simulink model "generate_elbow_motion"  (R2020b)
settings: Solver=FixedStepDiscrete  StartTime=0.0  StopTime=inf  FixedStep=0.001  RelTol=1e-3  EnableMultiTasking=on
PreLoadFcn:
  | demos_common_configs();
libraries: franka_simulink_library_misc x5, franka_simulink_library x4, simulink x1
settings Model: SimulationMode=external  ExtModeTrigDuration=10000  Creator=vasi_ko  LastModifiedBy=kvasios
settings DataIOCC: LimitDataPoints=on  SaveFormat=Array  ReturnWorkspaceOutputs=off
settings OptimizationCC: DefaultParameterBehavior=Inlined  EnhancedBackFolding=on  PassReuseOutputArgsAs=Individual arguments  ZeroExternalMemoryAtStartup=off  ZeroInternalMemoryAtStartup=off  OptimizeBlockOrder=speed  DifferentSizesBufferReuse=on  OptimizationCustomize=off  EfficientTunableParamExpr=on
settings DebuggingCC: SolverPrmCheckMsg=warning  ParameterTunabilityLossMsg=error  SFUnexpectedBacktrackingDiag=warning  SFNoUnconditionalDefaultTransitionDiag=warning  SFExecutionAtInitializationDiag=none  ArithmeticOperatorsInVariantConditions=warning
settings HardwareCC: ProdBitPerLong=64  ProdHWDeviceType=Intel->x86-64 (Linux 64)
settings ModelReferenceCC: PropagateSignalLabelsOutOfModel=off
settings SFSimCC: SimUseLocalCustomCode=off  MATLABDynamicMemAlloc=off  CustomCodeUndefinedFunction=UseInterfaceOnly  SimTargetLang=C++
settings RTWCC: Description=Embedded Coder  SystemTargetFile=franka_emika_panda.tlc  GenCodeOnly=on  TemplateMakefile=ert_default_tmf  RTWVerbose=off  RTWUseLocalCustomCode=off  Toolchain=Franka Simulink | gmake (64-bit linux)  BuildConfiguration=Faster Runs  IncludeHyperlinkInReport=on  TargetLang=C++
settings CodeAppCC: ForceParamTrailComments=on  IgnoreCustomStorageClasses=off  OperatorAnnotations=on  SimulinkDataObjDesc=on  SFDataObjDesc=on  InsertBlockDesc=on
settings STFCustomTargetCC: TargetLangStandard=C99 (ISO)  MultiwordLength=256  GenerateSampleERTMain=on  ModelReferenceCompliant=off  ConcurrentExecutionCompliant=off  CombineOutputUpdateFcns=on  ERTCustomFileBanners=on  SupportNonInlinedSFcns=off  RemoveResetFunc=on  MATLABClassNameForMDSCustomization=Simulink.SoftwareTarget.ERTCustomization  GRTInterface=off  UseToolchainInfoCompliant=on  SystemTargetFile=franka_emika_panda.tlc
settings ERTTargetCC: TargetLangStandard=C99 (ISO)  GenerateSampleERTMain=on  ModelReferenceCompliant=off  ParMdlRefBuildCompliant=off  CompOptLevelCompliant=off  ConcurrentExecutionCompliant=off  SupportContinuousTime=on  ModelStepFunctionPrototypeControlCompliant=off  InlinedParameterPlacement=NonHierarchical  ERTCustomFileTemplate=franka_emika_panda_file_process.tlc
settings ConfigComp: CovMetricSettings=dw  CovSaveCumulativeToWorkspaceVar=on  CovSaveSingleToWorkspaceVar=on  CovExternalEMLEnable=off  CovSFcnEnable=off

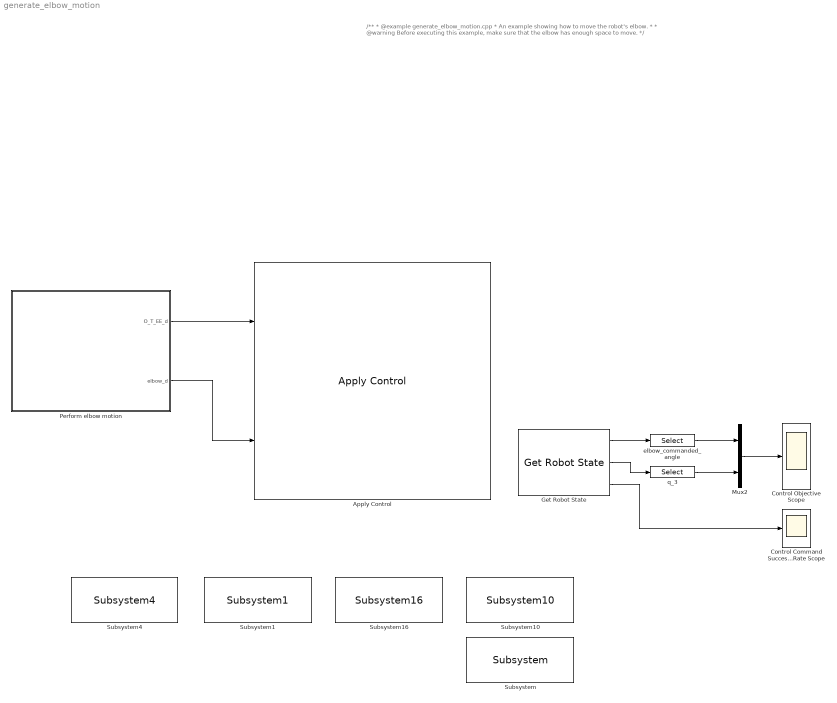
== system generate_elbow_motion ==
  note: /**
      |  * @example generate_elbow_motion.cpp
      |  * An example showing how to move the robot's elbow.
      |  *
      |  * @warning Before executing this example, make sure that the elbow has enough space to move.
      |  */
  Apply Control : franka_simulink_library/Apply Control  robot_ip=robot_ip  gripper_attached=off  control_mode=Cartesian Pose - Internal Controller Mode  controller_choice=Joint Impedance Controller  elbow_control=on  collision_thresholds=[25.0, 25.0, 22.0, 20.0, 19.0, 17.0, 14.0,35.0, 35.0, 32.0, 30.0, 29.0, 27.0, 24.0,25.0, 25.0, 22.0, 20.0, 19.0, 17.0, 14.0,35.0, 35.0, 32.0, 30.0, 29.0, 27.0, 24.0,30.0, 30.0, 30.0, 25.0, 25.0, 25.0,40.0, 40.0, 40.0, 35.0, 35.0, 35.0,30.0, 30.0, 30.0, 25.0, 25.0, 25.0,40.0, 40.0, 40.0, 35.0, 35.0, 35.0]  joint_impedance=[3000, 3000, 3000, 2500, 2500, 2000, 2000]  cartesian_impedance=cartesian_impedance  load_inertia=load_inertia  EE_T_K=EE_T_K  init_joint_configuration_req=on  init_joint_configuration=q_init
      settings: SourceProductName=Franka Emika
  Control Command Success Rate Scope : Scope
  Control Objective Scope : Scope
  Get Robot State : franka_simulink_library/Get Robot State  robot_ip=robot_ip  signals_requested='elbow_c q control_command_success_rate'
      settings: SourceProductName=Franka Emika
  Mux2 : Mux  Inputs=2
  Perform elbow motion : Subsystem
      mask Display:
      | pos = get_param(gcb, 'Position');
      | width = pos(3) - pos(1);
      | x = [0:width];
      | y = sin(x/180*pi);
      | % Parameters 'm' and 'b' must be defined in 'Parameters & Dialog' pane.
      | plot(cos(x/180*pi*0.5), sin(x/180*pi*0.5));
      | 
      | port_label('output',1,'O_T_EE_d');
      | port_label('output',2,'elbow_d');
  Subsystem : franka_simulink_library_misc/Subsystem  SystemSampleTime=-1  VariantActivationTime=update diagram  Latency=0  AutoFrameSizeCalculation=off
  Subsystem1 : franka_simulink_library_misc/Subsystem1  SystemSampleTime=-1  VariantActivationTime=update diagram  Latency=0  AutoFrameSizeCalculation=off
  Subsystem10 : franka_simulink_library_misc/Subsystem10  SystemSampleTime=-1  VariantActivationTime=update diagram  Latency=0  AutoFrameSizeCalculation=off
  Subsystem16 : franka_simulink_library_misc/Subsystem16  SystemSampleTime=-1  VariantActivationTime=update diagram  Latency=0  AutoFrameSizeCalculation=off
  Subsystem4 : franka_simulink_library_misc/Subsystem4  SystemSampleTime=-1  VariantActivationTime=update diagram  Latency=0  AutoFrameSizeCalculation=off
  elbow_commanded_angle : Selector  InputPortWidth=2  IndexOptions=Index vector (dialog)  Indices=1  OutputSizes=1
  q_3 : Selector  InputPortWidth=7  IndexOptions=Index vector (dialog)  Indices=3  OutputSizes=1
  wires:
  Perform elbow motion/1(O_T_EE_d) -> Apply Control/1
  Perform elbow motion/2(elbow_d) -> Apply Control/2
  Get Robot State/1 -> elbow_commanded_angle/1
  Get Robot State/2 -> q_3/1
  Mux2/1 -> Control Objective Scope/1
  elbow_commanded_angle/1 -> Mux2/1
  q_3/1 -> Mux2/2
  Get Robot State/3 -> Control Command Success Rate Scope/1

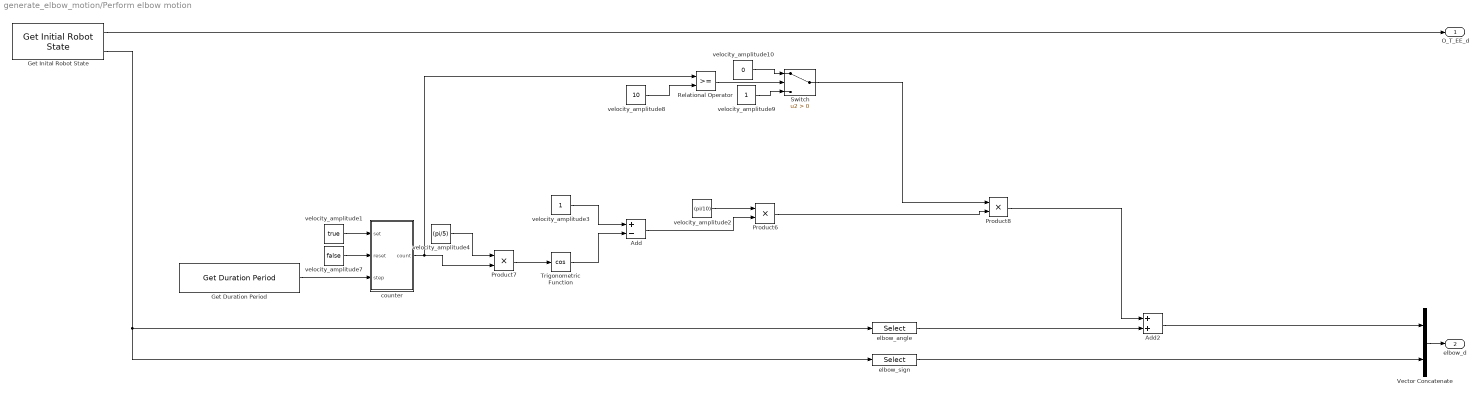
== system generate_elbow_motion/Perform elbow motion ==
  Add : Sum  Inputs=+-
  Add2 : Sum
  Get Duration Period : franka_simulink_library/Get Duration Period  robot_ip=robot_ip
      settings: SourceProductName=Franka Emika
  Get Inital Robot State : franka_simulink_library/Get Initial Robot State  robot_ip=robot_ip  signals_requested='O_T_EE_c elbow_c'
      settings: SourceProductName=Franka Emika
  Product6 : Product
  Product7 : Product
  Product8 : Product
  Relational Operator : RelationalOperator  OutDataTypeStr=boolean  RndMeth=Nearest
  Switch : Switch  Criteria=u2 > Threshold
  Trigonometric Function : Trigonometry  Operator=cos  NumberOfIterations=50
  Vector Concatenate : Concatenate
  counter : Subsystem
  elbow_angle : Selector  InputPortWidth=2  IndexOptions=Index vector (dialog)  Indices=1  OutputSizes=1
  elbow_sign : Selector  InputPortWidth=2  IndexOptions=Index vector (dialog)  Indices=2  OutputSizes=1
  velocity_amplitude1 : Constant  Value=true  VectorParams1D=off
  velocity_amplitude10 : Constant  Value=0  VectorParams1D=off
  velocity_amplitude2 : Constant  Value=(pi/10)  VectorParams1D=off
  velocity_amplitude3 : Constant  VectorParams1D=off
  velocity_amplitude4 : Constant  Value=(pi/5)  VectorParams1D=off
  velocity_amplitude7 : Constant  Value=false  VectorParams1D=off
  velocity_amplitude8 : Constant  Value=10  VectorParams1D=off
  velocity_amplitude9 : Constant  VectorParams1D=off
  O_T_EE_d : Outport  VectorParamsAs1DForOutWhenUnconnected=off
  elbow_d : Outport  Port=2  VectorParamsAs1DForOutWhenUnconnected=off
  wires:
  Product8/1 -> Add2/1
  elbow_angle/1 -> Add2/2
  Get Inital Robot State/2 -> elbow_angle/1, elbow_sign/1
  velocity_amplitude2/1 -> Product6/1
  velocity_amplitude3/1 -> Add/1
  velocity_amplitude4/1 -> Product7/1
  Trigonometric Function/1 -> Add/2
  Product7/1 -> Trigonometric Function/1
  Add/1 -> Product6/2
  Switch/1 -> Product8/1
  Get Duration Period/1 -> counter/3(step)
  velocity_amplitude1/1 -> counter/1(set)
  velocity_amplitude7/1 -> counter/2(reset)
  counter/1(count) -> Relational Operator/1, Product7/2
  velocity_amplitude8/1 -> Relational Operator/2
  Relational Operator/1 -> Switch/2
  velocity_amplitude9/1 -> Switch/3
  velocity_amplitude10/1 -> Switch/1
  Get Inital Robot State/1 -> O_T_EE_d/1
  Vector Concatenate/1 -> elbow_d/1
  Add2/1 -> Vector Concatenate/1
  elbow_sign/1 -> Vector Concatenate/2
  Product6/1 -> Product8/2

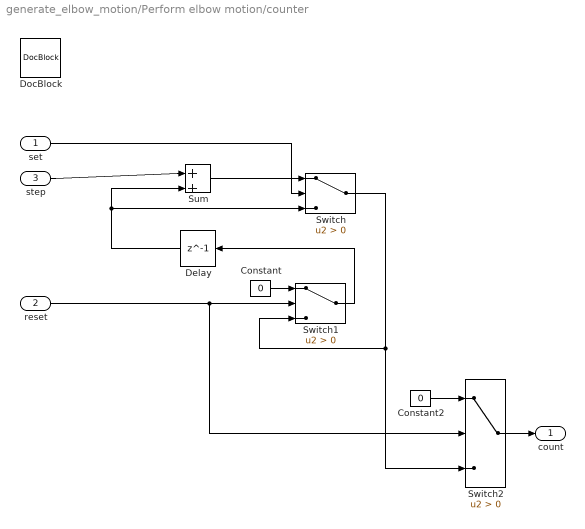
== system generate_elbow_motion/Perform elbow motion/counter ==
  set : Inport  OutDataTypeStr=boolean
  reset : Inport  Port=2  OutDataTypeStr=boolean
  step : Inport  Port=3  OutDataTypeStr=double
  Constant : Constant  Value=0  OutDataTypeStr=double
  Constant2 : Constant  Value=0  OutDataTypeStr=double
  Delay : Delay  DelayLength=1  InitialCondition=0
  DocBlock : simulink/Model-Wide Utilities/DocBlock  DocumentType=Text
      content=|
      | %% counter
      | %
      | % This library includes the counter functionality that increases
      | % it's output by an input step factor for each computational step. The counter
      | % can also be externaly reset.
      | % -----------------------------------------------------------------------
      | % Author    : Konstantinos Vasios
      | % Date      : 01.09.2017
      | % Copyright : Franka Emika GmbH
      | % -----------------------------------------------------------------------
      | %
      | % Inputs:
      | % @param set : activates the counter. (data type: boolean, dimension: 1)
      | % @param reset: it resets the counter. Count starts from 0. (data type: boolean, dimension: 1)
      | % @param step: increment factor. (data type: real, dimension: 1)
      | %
      | % Outputs:
      | % @return count: current counter value. (data type: real, dimension: 1)
      | %% -----------------------------------------------------------------------
  Sum : Sum  Inputs=|++
  Switch : Switch  Criteria=u2 > Threshold
  Switch1 : Switch  Criteria=u2 > Threshold  OutDataTypeStr=double
  Switch2 : Switch  Criteria=u2 > Threshold  OutDataTypeStr=double
  count : Outport  OutDataTypeStr=double  VectorParamsAs1DForOutWhenUnconnected=off
  wires:
  Switch1/1 -> Delay/1
  Constant/1 -> Switch1/1
  reset/1 -> Switch2/2, Switch1/2
  Delay/1 -> Switch/3, Sum/2
  step/1 -> Sum/1
  Switch/1 -> Switch2/3, Switch1/3
  set/1 -> Switch/2
  Sum/1 -> Switch/1
  Constant2/1 -> Switch2/1
  Switch2/1 -> count/1
